simulink model "Arm_Testing"  (R2023b)
settings: Solver=VariableStepAuto  StartTime=0.0  StopTime=10.0  FixedStep=0.02  MaxStep=0.02  RelTol=1e-3
undefined symbols (not defined in the file): Back_AA_Bot_Min_Ext, Back_AA_Top_Min_Ext, Dist_Per_Rev_Back_Lower
settings Model: Creator=ander  LastModifiedBy=ander

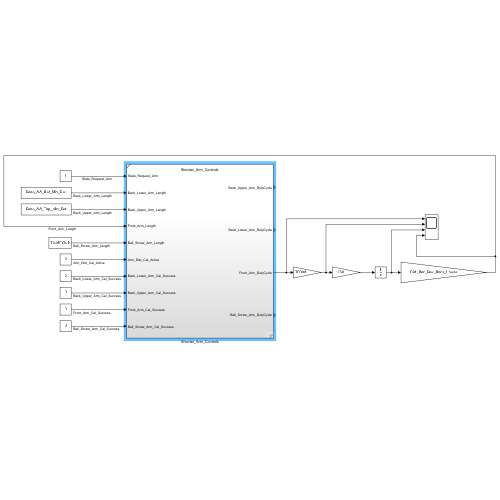
[thumbnail: Simulink's stored preview of the top-level diagram]
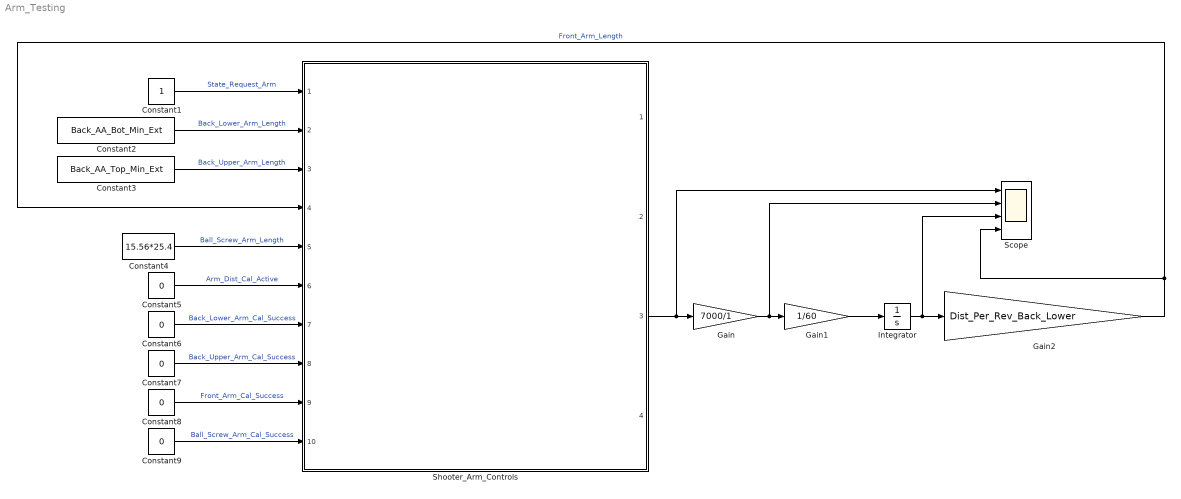
== system Arm_Testing ==
  Constant1 : Constant
  Constant2 : Constant  Value=Back_AA_Bot_Min_Ext
  Constant3 : Constant  Value=Back_AA_Top_Min_Ext
  Constant4 : Constant  Value=15.56*25.4
  Constant{5..9} (5 alike) : Constant  Value=0
  Gain : Gain  Gain=7000/1
  Gain1 : Gain  Gain=1/60
  Gain2 : Gain  Gain=Dist_Per_Rev_Back_Lower
  Integrator : Integrator
  Scope : Scope  NumInputPorts=4
  Shooter_Arm_Controls : Subsystem  ReferencedSubsystem=Shooter_Arm_Controls
  wires:
  Gain/1 -> Scope/2, Gain1/1
  Gain1/1 -> Integrator/1
  Integrator/1 -> Scope/3, Gain2/1
  Shooter_Arm_Controls/3 -> Scope/1, Gain/1
  Gain2/1 -> Scope/4, Shooter_Arm_Controls/4  "Front_Arm_Length"
  Constant1/1 -> Shooter_Arm_Controls/1  "State_Request_Arm"
  Constant2/1 -> Shooter_Arm_Controls/2  "Back_Lower_Arm_Length"
  Constant3/1 -> Shooter_Arm_Controls/3  "Back_Upper_Arm_Length"
  Constant4/1 -> Shooter_Arm_Controls/5  "Ball_Screw_Arm_Length"
  Constant5/1 -> Shooter_Arm_Controls/6  "Arm_Dist_Cal_Active"
  Constant6/1 -> Shooter_Arm_Controls/7  "Back_Lower_Arm_Cal_Success"
  Constant7/1 -> Shooter_Arm_Controls/8  "Back_Upper_Arm_Cal_Success"
  Constant8/1 -> Shooter_Arm_Controls/9  "Front_Arm_Cal_Success"
  Constant9/1 -> Shooter_Arm_Controls/10  "Ball_Screw_Arm_Cal_Success"
